simulink model "simulateDSSS_codeMultiplexing_withTS"  (R2017a)
settings: Solver=VariableStepAuto  StartTime=0.0  StopTime=10  RelTol=1e-3
InitFcn:
  | fs = 10e3;
  | Ts = 1/fs;
  | Tb = 0.1;
  | Tc = 0.0125;
  | frameSize = 1000;
libraries: commfilt2 x8, dspsrcs4 x4, commdigbbndpm3 x2, commrandsrc3 x2, commchan3 x1
settings Model: Creator=prust  LastModifiedBy=prust

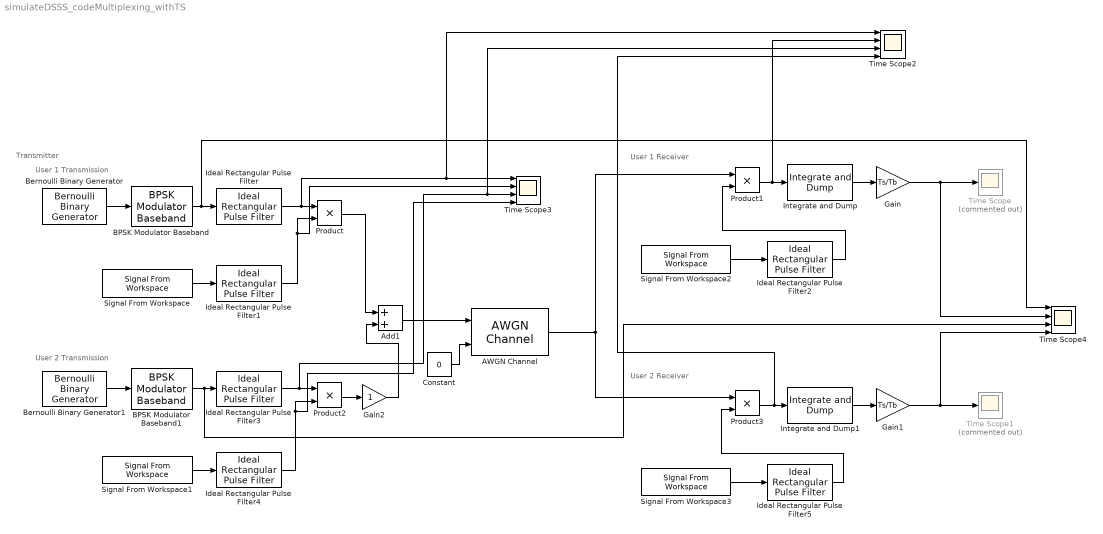
== system simulateDSSS_codeMultiplexing_withTS ==
  note: User 1 Receiver
  note: User 1 Transmission
  note: Transmitter
  note: User 2 Transmission
  note: User 2 Receiver
  AWGN Channel : commchan3/AWGN Channel  InputProcessing=Columns as channels (frame based)  seed=67  noiseMode=Variance from port  EbNodB=10  EsNodB=10  SNRdB=10  bitsPerSym=1  Ps=1  Tsym=1  variance=1
  Add1 : Sum
  BPSK Modulator Baseband : commdigbbndpm3/BPSK Modulator Baseband  Ph=0  outDtype=double  outWordLen=16  outUDDataType=sfix(16)  outFracLenMode=Best precision  outFracLen=15  outDataTypeStr=double  outLastDataTypeStr=double
  BPSK Modulator Baseband1 : commdigbbndpm3/BPSK Modulator Baseband  Ph=0  outDtype=double  outWordLen=16  outUDDataType=sfix(16)  outFracLenMode=Best precision  outFracLen=15  outDataTypeStr=double  outLastDataTypeStr=double
  Bernoulli Binary Generator : commrandsrc3/Bernoulli Binary Generator  ProbabilityOfZero=0.5  SeedSource=Auto  Seed=0  SampleTime=Tb  SamplesPerFrame=frameSize  OutputDataType=double  SimulateUsing=Interpreted execution
  Bernoulli Binary Generator1 : commrandsrc3/Bernoulli Binary Generator  ProbabilityOfZero=0.5  SeedSource=Auto  Seed=0  SampleTime=Tb  SamplesPerFrame=frameSize  OutputDataType=double  SimulateUsing=Interpreted execution
  Constant : Constant  Value=0
  Gain : Gain  Gain=Ts/Tb
  Gain1 : Gain  Gain=Ts/Tb
  Gain2 : Gain
  Ideal Rectangular Pulse Filter : commfilt2/Ideal Rectangular Pulse Filter  pulseLen=Tb/Ts  pulseDelay=0  InputProcessing=Columns as channels (frame based)  RateOptions=Allow multirate processing  sampMode=Mute  normCheck=off  normMode=Sum of samples  filterGain=1  saveAsFlag=0  roundingMode=Floor  overflowMode=off  firstCoeffDataTypeStr=Inherit: Same word length as input  firstCoeffMin=[]  firstCoeffMax=[]  firstCoeffLastDataTypeStr=Inherit: Same word length as input  outputDataTypeStr=Inherit: Same as accumulator  outputMin=[]  outputMax=[]  outputLastDataTypeStr=Inherit: Same as accumulator
      settings: SourceProductName=Communications System Toolbox  SourceProductBaseCode=CM
  Ideal Rectangular Pulse Filter{1..2,4..5} (4 alike) : commfilt2/Ideal Rectangular Pulse Filter  pulseLen=Tc/Ts  pulseDelay=0  InputProcessing=Columns as channels (frame based)  RateOptions=Allow multirate processing  sampMode=Mute  normCheck=off  normMode=Sum of samples  filterGain=1  saveAsFlag=0  roundingMode=Floor  overflowMode=off  firstCoeffDataTypeStr=Inherit: Same word length as input  firstCoeffMin=[]  firstCoeffMax=[]  firstCoeffLastDataTypeStr=Inherit: Same word length as input  outputDataTypeStr=Inherit: Same as accumulator  outputMin=[]  outputMax=[]  outputLastDataTypeStr=Inherit: Same as accumulator
      settings: SourceProductName=Communications System Toolbox  SourceProductBaseCode=CM
  Ideal Rectangular Pulse Filter3 : commfilt2/Ideal Rectangular Pulse Filter  pulseLen=Tb/Ts  pulseDelay=0  InputProcessing=Columns as channels (frame based)  RateOptions=Allow multirate processing  sampMode=Mute  normCheck=off  normMode=Sum of samples  filterGain=1  saveAsFlag=0  roundingMode=Floor  overflowMode=off  firstCoeffDataTypeStr=Inherit: Same word length as input  firstCoeffMin=[]  firstCoeffMax=[]  firstCoeffLastDataTypeStr=Inherit: Same word length as input  outputDataTypeStr=Inherit: Same as accumulator  outputMin=[]  outputMax=[]  outputLastDataTypeStr=Inherit: Same as accumulator
      settings: SourceProductName=Communications System Toolbox  SourceProductBaseCode=CM
  Integrate and Dump : commfilt2/Integrate and Dump  obssamples=Tb/Ts  offsetsamples=0  nodump=off  roundingMode=Floor  overflowMode=off  outputDataTypeStr=Inherit: Same as accumulator  outputLastDataTypeStr=Inherit: Same as accumulator
      settings: SourceProductName=Communications System Toolbox
  Integrate and Dump1 : commfilt2/Integrate and Dump  obssamples=Tb/Ts  offsetsamples=0  nodump=off  roundingMode=Floor  overflowMode=off  outputDataTypeStr=Inherit: Same as accumulator  outputLastDataTypeStr=Inherit: Same as accumulator
      settings: SourceProductName=Communications System Toolbox
  Product{,1..3} (4 alike) : Product
  Signal From Workspace : dspsrcs4/Signal From Workspace  X=[1 -1 -1 1 -1 1 1 -1]  Ts=Tc  nsamps=frameSize  OutputAfterFinalValue=Cyclic repetition  ignoreOrWarnInputAndFrameLengths=off  OutputFrames=off
  Signal From Workspace1 : dspsrcs4/Signal From Workspace  X=[1 1 -1 -1 1 1 -1 -1]  Ts=Tc  nsamps=frameSize  OutputAfterFinalValue=Cyclic repetition  ignoreOrWarnInputAndFrameLengths=off  OutputFrames=off
  Signal From Workspace2 : dspsrcs4/Signal From Workspace  X=[1 -1 -1 1 -1 1 1 -1]  Ts=Tc  nsamps=frameSize  OutputAfterFinalValue=Cyclic repetition  ignoreOrWarnInputAndFrameLengths=off  OutputFrames=off
  Signal From Workspace3 : dspsrcs4/Signal From Workspace  X=[1 1 1 1 1 1 1 1]  Ts=Tc  nsamps=frameSize  OutputAfterFinalValue=Cyclic repetition  ignoreOrWarnInputAndFrameLengths=off  OutputFrames=off
  Time Scope : Scope  Commented=on
  Time Scope1 : Scope  Commented=on
  Time Scope2 : Scope  NumInputPorts=4
  Time Scope3 : Scope  NumInputPorts=4
  Time Scope4 : Scope  NumInputPorts=4
  wires:
  Bernoulli Binary Generator/1 -> BPSK Modulator Baseband/1
  Ideal Rectangular Pulse Filter/1 -> Time Scope2/1, Time Scope3/1, Product/1
  Signal From Workspace/1 -> Ideal Rectangular Pulse Filter1/1
  Ideal Rectangular Pulse Filter1/1 -> Time Scope3/2, Product/2
  Add1/1 -> AWGN Channel/1
  Constant/1 -> AWGN Channel/2
  Product/1 -> Add1/1
  Signal From Workspace2/1 -> Ideal Rectangular Pulse Filter2/1
  Ideal Rectangular Pulse Filter2/1 -> Product1/2
  AWGN Channel/1 -> Product3/1, Product1/1
  Product1/1 -> Time Scope2/2, Integrate and Dump/1
  Signal From Workspace1/1 -> Ideal Rectangular Pulse Filter4/1
  Ideal Rectangular Pulse Filter4/1 -> Time Scope3/4, Product2/2
  Ideal Rectangular Pulse Filter3/1 -> Time Scope2/3, Time Scope3/3, Product2/1
  Integrate and Dump/1 -> Gain/1
  Product2/1 -> Gain2/1
  Bernoulli Binary Generator1/1 -> BPSK Modulator Baseband1/1
  BPSK Modulator Baseband/1 -> Time Scope4/1, Ideal Rectangular Pulse Filter/1
  BPSK Modulator Baseband1/1 -> Time Scope4/3, Ideal Rectangular Pulse Filter3/1
  Gain/1 -> Time Scope4/2, Time Scope/1
  Signal From Workspace3/1 -> Ideal Rectangular Pulse Filter5/1
  Ideal Rectangular Pulse Filter5/1 -> Product3/2
  Product3/1 -> Time Scope2/4, Integrate and Dump1/1
  Integrate and Dump1/1 -> Gain1/1
  Gain1/1 -> Time Scope4/4, Time Scope1/1
  Gain2/1 -> Add1/2
